simulink model "state_spacemodel"  (R2017b)
settings: Solver=VariableStepAuto  StartTime=0.0  StopTime=inf  RelTol=1e-3
values from neighbouring files (symbols this model uses):
  A = A'    [c_l.m]    (also in c_m.m; c_n.m; c_x.m; c_z.m)
  B = ssm_b( state_trim, state_dot_trim, control_trim, xcg )    [ssm_f16.m]    (also in thrust.m = B')
  C = ssm_c( state_trim, state_dot_trim, control_trim, xcg )    [ssm_f16.m]    (also in thrust.m = C')
  control_trim = u0    [find_trim.m]
  D = ssm_d( state_trim, state_dot_trim, control_trim, xcg )    [ssm_f16.m]
  trim_control = [UX(2);UX(4);UX(5)]    [trim_F16.m]
  trim_state = xu(1:12)    [trim_F16.m]
  trim_thrust = UX(1)    [trim_F16.m]
libraries: simulink x3
settings Model: Creator=monster  LastModifiedBy=monster

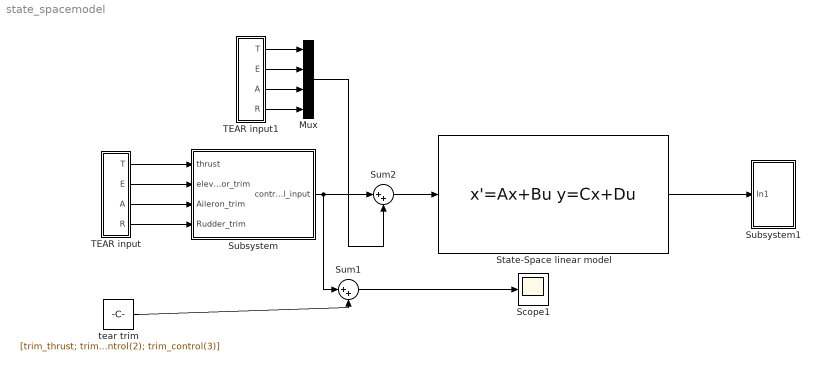
== system state_spacemodel ==
  Mux : Mux
  Scope1 : Scope
  "State-Space linear model " : StateSpace  A=A  B=B  C=C  D=D  InitialCondition=[trim_state]
      mask Display: image('D:\Dropbox\M.eng\fall2017\flight control system\FDC\project\control surface.PNG');
  Subsystem : Subsystem
  Subsystem1 : Subsystem
  Sum1 : Sum  Inputs=|++  SaturateOnIntegerOverflow=on  InputSameDT=on  OutDataTypeStr=Inherit: Same as first input
  Sum2 : Sum  Inputs=|++  SaturateOnIntegerOverflow=on  InputSameDT=on  OutDataTypeStr=Inherit: Same as first input
  TEAR input : Subsystem
  TEAR input1 : Subsystem
  tear trim : Constant  Value=[trim_thrust; trim_control(1); trim_control(2); trim_control(3)]
  wires:
  TEAR input/4(R) -> Subsystem/4(Rudder_trim)
  TEAR input/3(A) -> Subsystem/3(Aileron_trim)
  TEAR input/2(E) -> Subsystem/2(elevator_trim)
  TEAR input/1(T) -> Subsystem/1(thrust)
  tear trim/1 -> Sum1/2
  Sum1/1 -> Scope1/1
  Subsystem/1(control_input) -> Sum2/1, Sum1/1
  "State-Space linear model "/1 -> Subsystem1/1(In1)
  TEAR input1/2(E) -> Mux/2
  TEAR input1/1(T) -> Mux/1
  TEAR input1/3(A) -> Mux/3
  TEAR input1/4(R) -> Mux/4
  Mux/1 -> Sum2/2
  Sum2/1 -> "State-Space linear model "/1

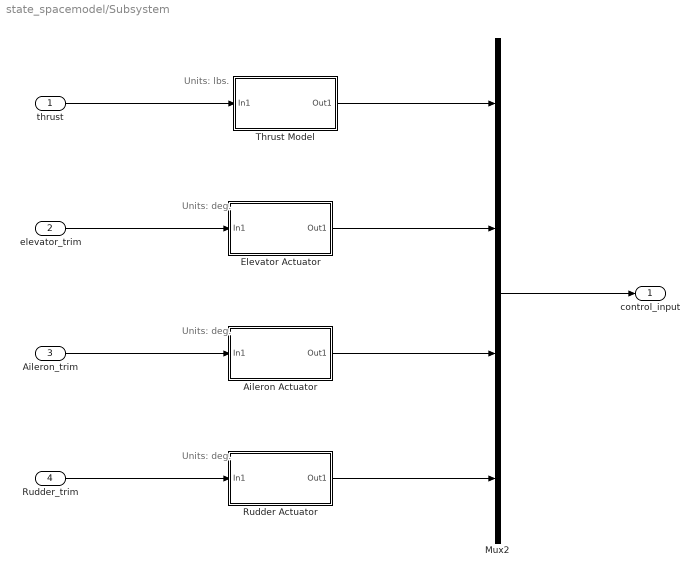
== system state_spacemodel/Subsystem ==
  note: Units: deg.
  note: Units: deg.
  note: Units: lbs.
  note: Units: deg.
  thrust : Inport
  elevator_trim : Inport  Port=2
  Aileron_trim : Inport  Port=3
  Rudder_trim : Inport  Port=4
  Aileron Actuator : Subsystem  AncestorBlock=F16_Actuator_Library/Aileron Actuator
  Elevator Actuator : Subsystem  AncestorBlock=F16_Actuator_Library/Elevator Actuator
  Mux2 : Mux
  Rudder Actuator : Subsystem  AncestorBlock=F16_Actuator_Library/Rudder Actuator
  Thrust Model : Subsystem  AncestorBlock=F16_Actuator_Library/Thrust Model
  control_input : Outport
  wires:
  thrust/1 -> Thrust Model/1(In1)
  Aileron Actuator/1(Out1) -> Mux2/3
  Rudder_trim/1 -> Rudder Actuator/1(In1)
  Elevator Actuator/1(Out1) -> Mux2/2
  Rudder Actuator/1(Out1) -> Mux2/4
  elevator_trim/1 -> Elevator Actuator/1(In1)
  Aileron_trim/1 -> Aileron Actuator/1(In1)
  Thrust Model/1(Out1) -> Mux2/1
  Mux2/1 -> control_input/1

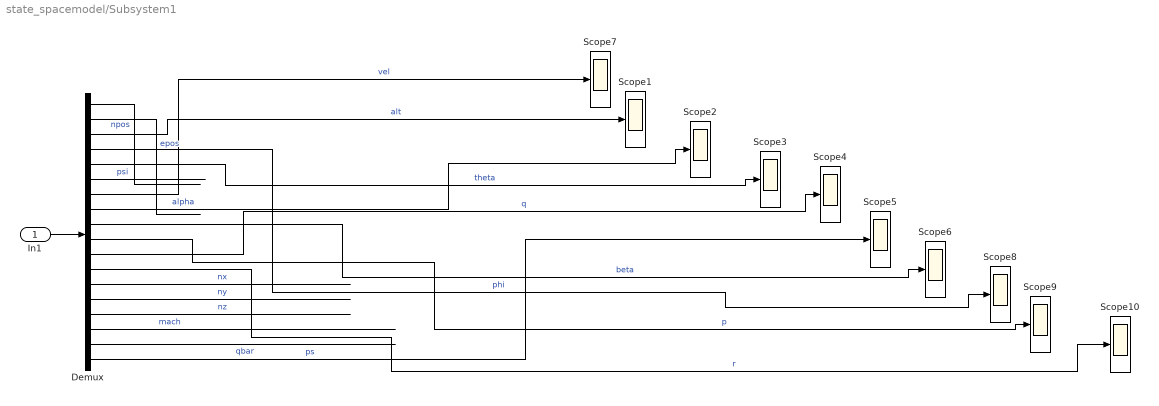
== system state_spacemodel/Subsystem1 ==
  In1 : Inport
  Demux : Demux  Outputs=18
  Scope{1..10} (10 alike) : Scope
  wires:
  Demux/3 -> Scope1/1  "alt"
  Demux/4 -> Scope8/1  "phi"
  Demux/8 -> Scope2/1  "alpha"
  Demux/13 -> ?  "nx"
  Demux/2 -> ?  "epos"
  Demux/10 -> Scope9/1  "p"
  Demux/6 -> ?  "psi"
  Demux/18 -> Scope5/1  "ps"
  Demux/16 -> ?  "mach"
  Demux/15 -> ?  "nz"
  Demux/1 -> ?  "npos"
  Demux/5 -> Scope3/1  "theta"
  Demux/7 -> Scope7/1  "vel"
  Demux/14 -> ?  "ny"
  Demux/12 -> Scope10/1  "r"
  Demux/17 -> ?  "qbar"
  Demux/9 -> Scope6/1  "beta"
  Demux/11 -> Scope4/1  "q"
  In1/1 -> Demux/1

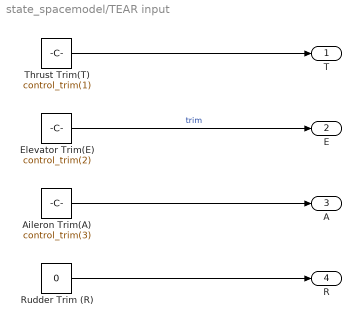
== system state_spacemodel/TEAR input ==
  "Aileron Trim(A) " : Constant  Value=control_trim(3)
  "Elevator Trim(E) " : Constant  Value=control_trim(2)  VectorParams1D=off
  Rudder Trim (R) : Constant  Value=0
  "Thrust Trim(T) " : Constant  Value=control_trim(1)
  T : Outport
  E : Outport  Port=2
  A : Outport  Port=3
  R : Outport  Port=4
  wires:
  "Aileron Trim(A) "/1 -> A/1
  "Elevator Trim(E) "/1 -> E/1  "trim"
  "Thrust Trim(T) "/1 -> T/1
  Rudder Trim (R)/1 -> R/1

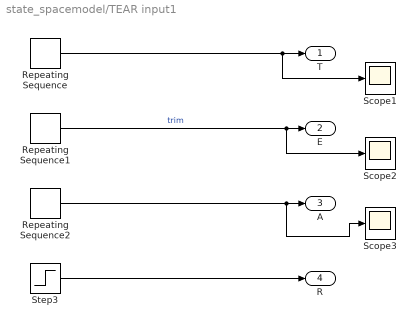
== system state_spacemodel/TEAR input1 ==
  Repeating Sequence : simulink/Sources/Repeating Sequence  rep_seq_t="[0 2 4 6 8 10 12 14 16 18 20  ]"  rep_seq_y="[0 -1000 0 0 0 0 0 0 0 0 0  ]"
  Repeating Sequence1 : simulink/Sources/Repeating Sequence  rep_seq_t="[0 2 4 6 8 10 12 14 16 18 20  ]"  rep_seq_y="[0 0 5 0 0 0 0 0 0 0 0  ]"
  Repeating Sequence2 : simulink/Sources/Repeating Sequence  rep_seq_t="[0 2 4 6 8 10 12 14 16 18 20  ]"  rep_seq_y="[0 0 0 5 0 0 0 0 0 0 0  ]"
  Scope1 : Scope
  Scope2 : Scope
  Scope3 : Scope
  Step3 : Step  After=0  SampleTime=0
  T : Outport
  E : Outport  Port=2
  A : Outport  Port=3
  R : Outport  Port=4
  wires:
  Repeating Sequence2/1 -> Scope3/1, A/1
  Repeating Sequence1/1 -> Scope2/1, E/1  "trim"
  Repeating Sequence/1 -> Scope1/1, T/1
  Step3/1 -> R/1

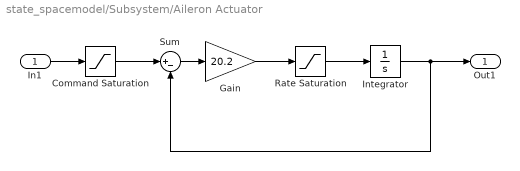
== system state_spacemodel/Subsystem/Aileron Actuator ==
  In1 : Inport
  Command Saturation : Saturate  UpperLimit=21.5  LowerLimit=-21.5
  Gain : Gain  Gain=20.2  SaturateOnIntegerOverflow=on  OutDataTypeStr=Inherit: Same as input  ParamDataTypeStr=Inherit: Same as input
  "Integrator " : Integrator  InitialCondition=control_trim(3)  UpperSaturationLimit=21.5  LowerSaturationLimit=-21.5
  Rate Saturation : Saturate  UpperLimit=80  LowerLimit=-80
  Sum : Sum  Inputs=|+-  SaturateOnIntegerOverflow=on  InputSameDT=on  OutDataTypeStr=Inherit: Same as first input
  Out1 : Outport
  wires:
  "Integrator "/1 -> Sum/2, Out1/1
  Rate Saturation/1 -> "Integrator "/1
  Gain/1 -> Rate Saturation/1
  Sum/1 -> Gain/1
  Command Saturation/1 -> Sum/1
  In1/1 -> Command Saturation/1

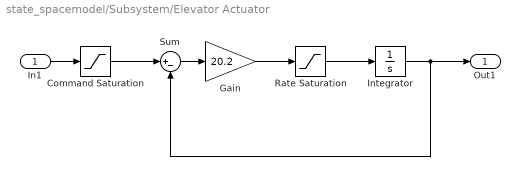
== system state_spacemodel/Subsystem/Elevator Actuator ==
  In1 : Inport
  Command Saturation : Saturate  UpperLimit=25  LowerLimit=-25
  Gain : Gain  Gain=20.2  SaturateOnIntegerOverflow=on  OutDataTypeStr=Inherit: Same as input  ParamDataTypeStr=Inherit: Same as input
  "Integrator " : Integrator  InitialCondition=control_trim(2)  UpperSaturationLimit=25  LowerSaturationLimit=-25
  Rate Saturation : Saturate  UpperLimit=60  LowerLimit=-60
  Sum : Sum  Inputs=|+-  SaturateOnIntegerOverflow=on  InputSameDT=on  OutDataTypeStr=Inherit: Same as first input
  Out1 : Outport
  wires:
  "Integrator "/1 -> Sum/2, Out1/1
  Rate Saturation/1 -> "Integrator "/1
  Gain/1 -> Rate Saturation/1
  Sum/1 -> Gain/1
  Command Saturation/1 -> Sum/1
  In1/1 -> Command Saturation/1

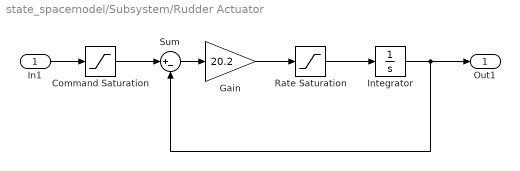
== system state_spacemodel/Subsystem/Rudder Actuator ==
  In1 : Inport
  Command Saturation : Saturate  UpperLimit=30  LowerLimit=-30
  Gain : Gain  Gain=20.2  SaturateOnIntegerOverflow=on  OutDataTypeStr=Inherit: Same as input  ParamDataTypeStr=Inherit: Same as input
  "Integrator " : Integrator  UpperSaturationLimit=30  LowerSaturationLimit=-30
  Rate Saturation : Saturate  UpperLimit=120  LowerLimit=-120
  Sum : Sum  Inputs=|+-  SaturateOnIntegerOverflow=on  InputSameDT=on  OutDataTypeStr=Inherit: Same as first input
  Out1 : Outport
  wires:
  "Integrator "/1 -> Sum/2, Out1/1
  Rate Saturation/1 -> "Integrator "/1
  Gain/1 -> Rate Saturation/1
  Sum/1 -> Gain/1
  Command Saturation/1 -> Sum/1
  In1/1 -> Command Saturation/1

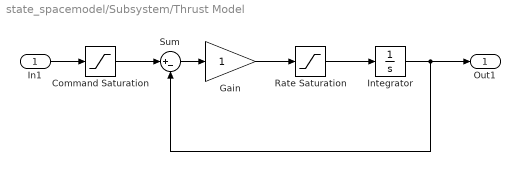
== system state_spacemodel/Subsystem/Thrust Model ==
  In1 : Inport
  Command Saturation : Saturate  UpperLimit=19000  LowerLimit=1000
  Gain : Gain  SaturateOnIntegerOverflow=on  OutDataTypeStr=Inherit: Same as input  ParamDataTypeStr=Inherit: Same as input
  "Integrator " : Integrator  InitialCondition=control_trim(1)  UpperSaturationLimit=30  LowerSaturationLimit=-30
  Rate Saturation : Saturate  UpperLimit=10000  LowerLimit=-10000
  Sum : Sum  Inputs=|+-  SaturateOnIntegerOverflow=on  InputSameDT=on  OutDataTypeStr=Inherit: Same as first input
  Out1 : Outport
  wires:
  "Integrator "/1 -> Sum/2, Out1/1
  Rate Saturation/1 -> "Integrator "/1
  Gain/1 -> Rate Saturation/1
  Sum/1 -> Gain/1
  Command Saturation/1 -> Sum/1
  In1/1 -> Command Saturation/1
